simulink model "Sim_LinearInvertedPendulum"  (R2022a)
settings: Solver=VariableStepAuto  StartTime=0.0  StopTime=5  RelTol=1e-3
undefined symbols (not defined in the file): A_disc, B_disc, K_Gains, Ts
settings Model: Creator=3060  LastModifiedBy=3060

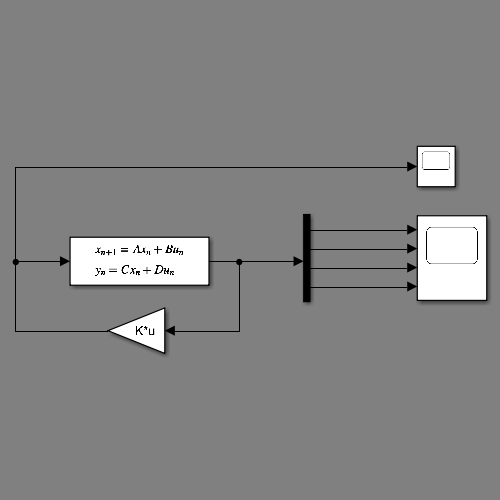
[thumbnail: Simulink's stored preview of the top-level diagram]
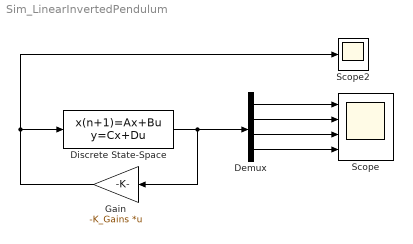
== system Sim_LinearInvertedPendulum ==
  Demux : Demux
  Discrete State-Space : DiscreteStateSpace  A=A_disc  B=B_disc  C=[1 0 0 0;0 1 0 0;0 0 1 0;0 0 0 1]  D=[0;0;0;0]  InitialCondition="[0, 0,  0.26, 0]"  SampleTime=Ts
  Gain : Gain  Gain=-K_Gains  Multiplication=Matrix(K*u)
  Scope : Scope  NumInputPorts=4
  Scope2 : Scope
  wires:
  Discrete State-Space/1 -> Gain/1, Demux/1
  Demux/1 -> Scope/1
  Demux/2 -> Scope/2
  Demux/3 -> Scope/3
  Demux/4 -> Scope/4
  Gain/1 -> Discrete State-Space/1, Scope2/1
